simulink model "model1"  (R2021b)
settings: Solver=VariableStepAuto  StartTime=0.0  StopTime=10.0  RelTol=1e-3
settings Model: Creator=Kirill  LastModifiedBy=Kirill
settings DebuggingCC: UnconnectedInputMsg=none  UnconnectedOutputMsg=none  UnconnectedLineMsg=none
settings RTWCC: DLArmComputeVersion=20.02.1

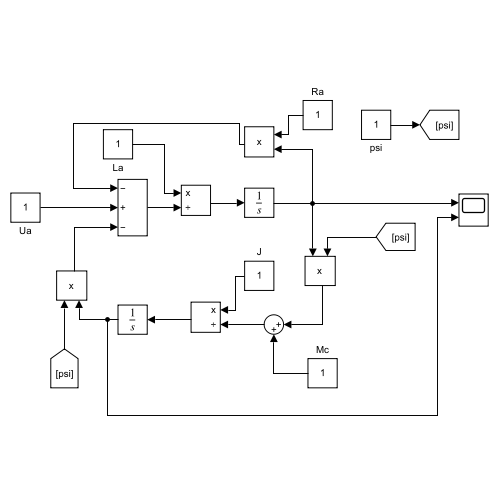
[thumbnail: Simulink's stored preview of the top-level diagram]
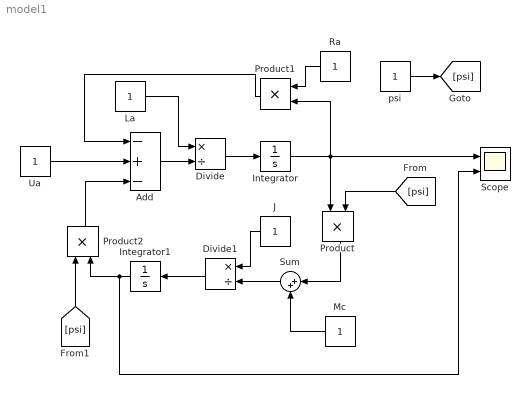
== system model1 ==
  Add : Sum  Inputs=-+-
  Divide : Product  Inputs=*/
  Divide1 : Product  Inputs=*/
  Integrator : Integrator
  Integrator1 : Integrator
  J : Constant
  La : Constant
  Mc : Constant
  Product : Product
  Product1 : Product
  Product2 : Product
  Ra : Constant
  Scope : Scope  NumInputPorts=2
  Sum : Sum  Inputs=|++
  Ua : Constant
  psi : Constant
  wires:
  Ua/1 -> Add/2
  Add/1 -> Divide/2
  Divide/1 -> Integrator/1
  Integrator/1 -> Scope/1, Product1/2, Product/1
  Ra/1 -> Product1/1
  Product1/1 -> Add/1
  psi/1 -> [psi]
  [psi] -> Product/2
  Product/1 -> Sum/1
  Mc/1 -> Sum/2
  Sum/1 -> Divide1/2
  J/1 -> Divide1/1
  Divide1/1 -> Integrator1/1
  Integrator1/1 -> Scope/2, Product2/2
  [psi] -> Product2/1
  Product2/1 -> Add/3
  La/1 -> Divide/1
